simulink model "Lab7_DIF"  (R2023b)
settings: Solver=VariableStepAuto  StartTime=0.0  StopTime=10.0  RelTol=1e-3
undefined symbols (not defined in the file or in its folder): i

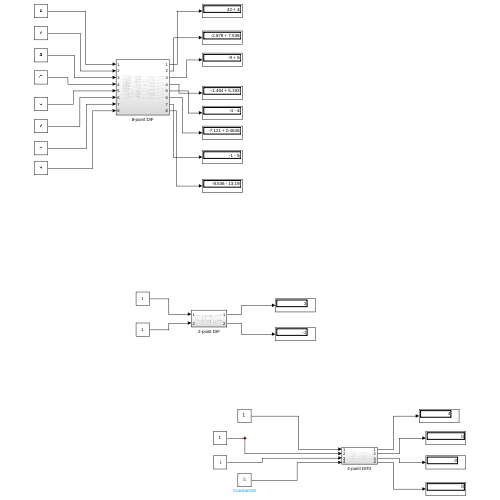
[thumbnail: Simulink's stored preview of the top-level diagram]
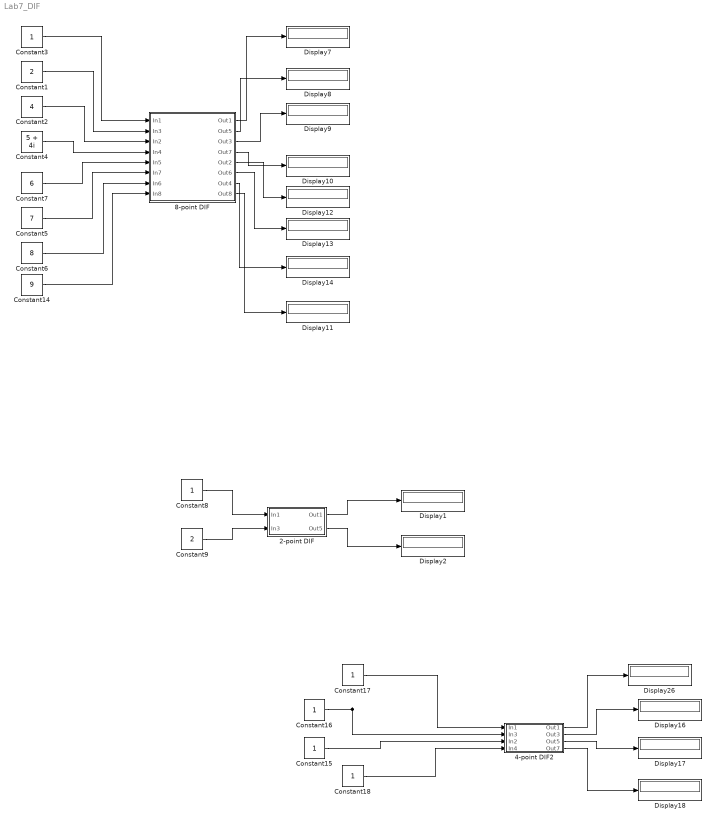
== system Lab7_DIF ==
  2-point DIF : Subsystem
  4-point DIF2 : Subsystem
  8-point DIF : Subsystem
  Constant1 : Constant  Value=2
  Constant14 : Constant  Value=9
  Constant{3,8,15..18} (6 alike) : Constant
  Constant2 : Constant  Value=4
  Constant4 : Constant  Value=5 + 4i
  Constant5 : Constant  Value=7
  Constant6 : Constant  Value=8
  Constant7 : Constant  Value=6
  Constant9 : Constant  Value=2
  Display{1..2,7..14,16..18,26} (14 alike) : Display
  wires:
  Constant8/1 -> 2-point DIF/1(In1)
  Constant9/1 -> 2-point DIF/2(In3)
  2-point DIF/2(Out5) -> Display2/1
  2-point DIF/1(Out1) -> Display1/1
  Constant3/1 -> 8-point DIF/1(In1)
  Constant1/1 -> 8-point DIF/2(In3)
  Constant2/1 -> 8-point DIF/3(In2)
  Constant4/1 -> 8-point DIF/4(In4)
  Constant7/1 -> 8-point DIF/5(In5)
  8-point DIF/1(Out1) -> Display7/1
  8-point DIF/2(Out5) -> Display8/1
  8-point DIF/3(Out3) -> Display9/1
  8-point DIF/4(Out7) -> Display10/1
  8-point DIF/5(Out2) -> Display12/1
  8-point DIF/6(Out6) -> Display13/1
  Constant5/1 -> 8-point DIF/6(In7)
  Constant6/1 -> 8-point DIF/7(In6)
  Constant14/1 -> 8-point DIF/8(In8)
  8-point DIF/7(Out4) -> Display14/1
  8-point DIF/8(Out8) -> Display11/1
  Constant15/1 -> 4-point DIF2/3(In2)
  Constant18/1 -> 4-point DIF2/4(In4)
  4-point DIF2/3(Out5) -> Display17/1
  4-point DIF2/2(Out3) -> Display16/1
  Constant16/1 -> 4-point DIF2/2(In3)
  4-point DIF2/4(Out7) -> Display18/1
  4-point DIF2/1(Out1) -> Display26/1
  Constant17/1 -> 4-point DIF2/1(In1)

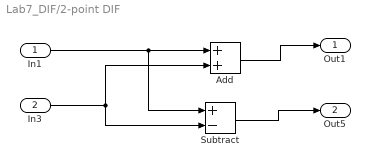
== system Lab7_DIF/2-point DIF ==
  In1 : Inport
  In3 : Inport  Port=2
  Add : Sum
  Subtract : Sum  Inputs=+-
  Out1 : Outport
  Out5 : Outport  Port=2
  wires:
  Add/1 -> Out1/1
  Subtract/1 -> Out5/1
  In1/1 -> Subtract/1, Add/1
  In3/1 -> Subtract/2, Add/2

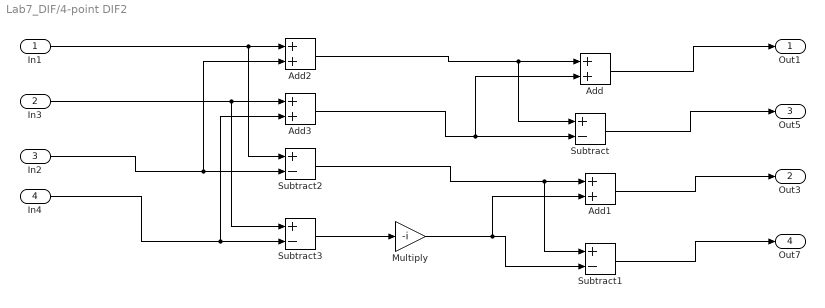
== system Lab7_DIF/4-point DIF2 ==
  In1 : Inport
  In3 : Inport  Port=2
  In2 : Inport  Port=3
  In4 : Inport  Port=4
  Add{,1..3} (4 alike) : Sum
  Multiply : Gain  Gain=-i
  Subtract{,1..3} (4 alike) : Sum  Inputs=+-
  Out1 : Outport
  Out3 : Outport  Port=2
  Out5 : Outport  Port=3
  Out7 : Outport  Port=4
  wires:
  Subtract3/1 -> Multiply/1
  Add/1 -> Out1/1
  Subtract/1 -> Out5/1
  Add1/1 -> Out3/1
  Subtract1/1 -> Out7/1
  In1/1 -> Subtract2/1, Add2/1
  In3/1 -> Subtract3/1, Add3/1
  In2/1 -> Add2/2, Subtract2/2
  In4/1 -> Add3/2, Subtract3/2
  Add2/1 -> Subtract/1, Add/1
  Add3/1 -> Add/2, Subtract/2
  Subtract2/1 -> Subtract1/1, Add1/1
  Multiply/1 -> Add1/2, Subtract1/2

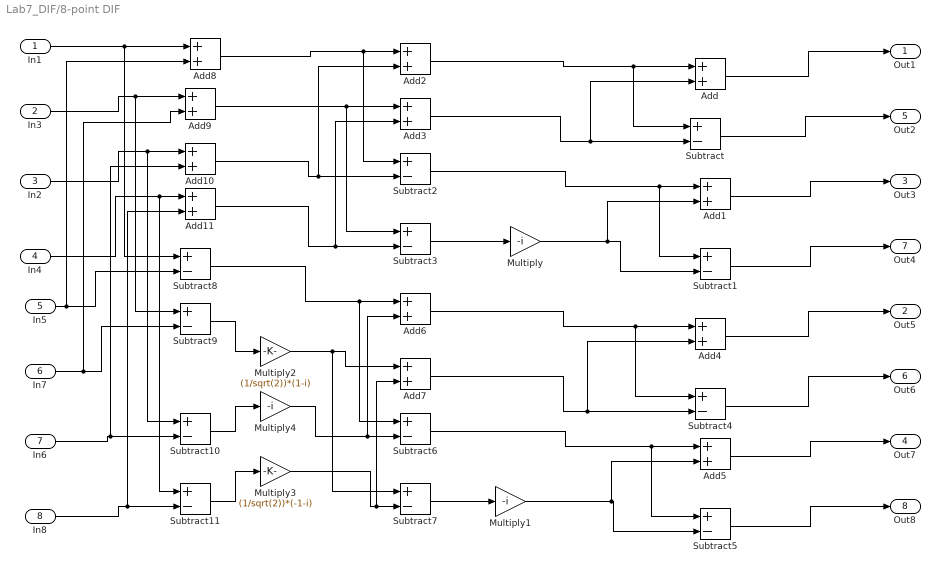
== system Lab7_DIF/8-point DIF ==
  In1 : Inport
  In3 : Inport  Port=2
  In2 : Inport  Port=3
  In4 : Inport  Port=4
  In5 : Inport  Port=5
  In7 : Inport  Port=6
  In6 : Inport  Port=7
  In8 : Inport  Port=8
  Add{,1..11} (12 alike) : Sum
  Multiply : Gain  Gain=-i
  Multiply1 : Gain  Gain=-i
  Multiply2 : Gain  Gain=(1/sqrt(2))*(1-i)
  Multiply3 : Gain  Gain=(1/sqrt(2))*(-1-i)
  Multiply4 : Gain  Gain=-i
  Subtract{,1..11} (12 alike) : Sum  Inputs=+-
  Out1 : Outport
  Out5 : Outport  Port=2
  Out3 : Outport  Port=3
  Out7 : Outport  Port=4
  Out2 : Outport  Port=5
  Out6 : Outport  Port=6
  Out4 : Outport  Port=7
  Out8 : Outport  Port=8
  wires:
  In1/1 -> Subtract8/1, Add8/1
  In3/1 -> Subtract9/1, Add9/1
  In2/1 -> Subtract10/1, Add10/1
  In4/1 -> Add11/1, Subtract11/1
  In8/1 -> Subtract11/2, Add11/2
  In6/1 -> Add10/2, Subtract10/2
  In7/1 -> Subtract9/2, Add9/2
  In5/1 -> Add8/2, Subtract8/2
  Subtract11/1 -> Multiply3/1
  Subtract10/1 -> Multiply4/1
  Subtract9/1 -> Multiply2/1
  Subtract7/1 -> Multiply1/1
  Subtract3/1 -> Multiply/1
  Add/1 -> Out1/1
  Subtract/1 -> Out2/1
  Add1/1 -> Out3/1
  Subtract1/1 -> Out4/1
  Add4/1 -> Out5/1
  Subtract4/1 -> Out6/1
  Add5/1 -> Out7/1
  Subtract5/1 -> Out8/1
  Add8/1 -> Subtract2/1, Add2/1
  Add9/1 -> Subtract3/1, Add3/1
  Add10/1 -> Add2/2, Subtract2/2
  Add11/1 -> Add3/2, Subtract3/2
  Subtract8/1 -> Subtract6/1, Add6/1
  Multiply2/1 -> Subtract7/1, Add7/1
  Multiply4/1 -> Add6/2, Subtract6/2
  Multiply3/1 -> Add7/2, Subtract7/2
  Add2/1 -> Subtract/1, Add/1
  Add3/1 -> Add/2, Subtract/2
  Subtract2/1 -> Subtract1/1, Add1/1
  Multiply/1 -> Add1/2, Subtract1/2
  Add6/1 -> Subtract4/1, Add4/1
  Add7/1 -> Add4/2, Subtract4/2
  Subtract6/1 -> Subtract5/1, Add5/1
  Multiply1/1 -> Add5/2, Subtract5/2
